simulink model "sol1"  (R2021b)
settings: Solver=VariableStepAuto  StartTime=0.0  StopTime=1  RelTol=1e-3
PreLoadFcn:
  | initModelData
values from neighbouring files (symbols this model uses):
  Bm = 4e-4    (= 0.0004)    [MyData_for_1_and_2.m]    (also in MyData_for_3_4_and_5.m; MyData_for_5_and_6.m)
  Jm = 5.5e-4    (= 0.00055)    [MyData_for_1_and_2.m]    (also in MyData_for_3_4_and_5.m; MyData_for_5_and_6.m)
  Kb = 0.105    [MyData_for_1_and_2.m]    (also in MyData_for_3_4_and_5.m; MyData_for_5_and_6.m)
  Km = 0.105    [MyData_for_1_and_2.m]    (also in MyData_for_3_4_and_5.m; MyData_for_5_and_6.m)
  L = 0.9e-3    (= 0.0009)    [MyData_for_1_and_2.m]    (also in MyData_for_3_4_and_5.m; MyData_for_5_and_6.m)
  r = 156    [MyData_for_1_and_2.m]    (also in MyData_for_3_4_and_5.m; MyData_for_5_and_6.m)
  R = 0.76    [MyData_for_1_and_2.m]    (also in MyData_for_3_4_and_5.m; MyData_for_5_and_6.m)
settings Model: Creator=esdan  LastModifiedBy=munir
settings SolverCC: AlgebraicLoopSolver=TrustRegion
settings DebuggingCC: SFMachineParentedDataDiag=warning

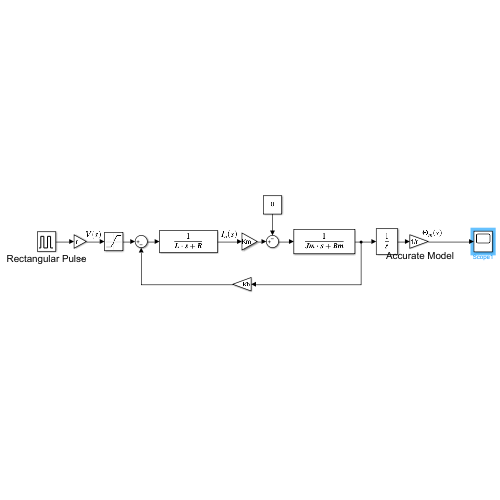
[thumbnail: Simulink's stored preview of the top-level diagram]
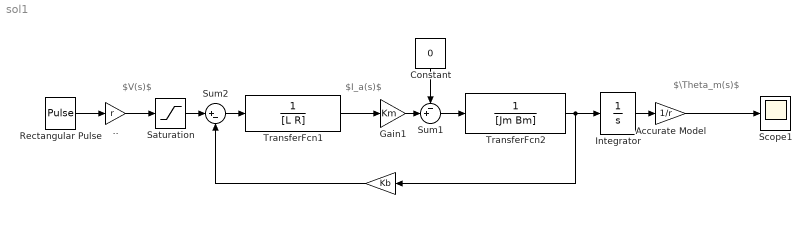
== system sol1 ==
  note: $I_a(s)$
  note: $\Theta_m(s)$
  note: $V(s)$
  " " : Gain  Gain=Kb
  " .." : Gain  Gain=r
  " Accurate Model" : Gain  Gain=1/r
  Constant : Constant  Value=0
  Gain1 : Gain  Gain=Km
  Integrator : Integrator
  Rectangular Pulse : DiscretePulseGenerator  PulseType=Time based  Period=1  PulseWidth=50
  Saturation : Saturate  UpperLimit=35  LowerLimit=-35
  Scope1 : Scope
  Sum1 : Sum  Inputs=-+|
  Sum2 : Sum  Inputs=|+-
  TransferFcn1 : TransferFcn  Denominator=[L R]
  TransferFcn2 : TransferFcn  Denominator=[Jm Bm]
  wires:
  TransferFcn1/1 -> Gain1/1
  Sum2/1 -> TransferFcn1/1
  TransferFcn2/1 -> " "/1, Integrator/1
  " "/1 -> Sum2/2
  Saturation/1 -> Sum2/1
  Sum1/1 -> TransferFcn2/1
  Gain1/1 -> Sum1/2
  Constant/1 -> Sum1/1
  " .."/1 -> Saturation/1
  " Accurate Model"/1 -> Scope1/1
  Integrator/1 -> " Accurate Model"/1
  Rectangular Pulse/1 -> " .."/1
